simulink model "SimuRISC"  (R2024b)
settings: Solver=FixedStepAuto  StartTime=0.0  StopTime=inf  RelTol=1e-3
values from neighbouring files (symbols this model uses):
  entryPointAddress = hex2dec('80000000')    [initSimuRISC.m]
  modelStopCondition = "tohost"    [initSimuRISC.m]
  tohost_address = hex2dec('1000')    [initSimuRISC.m]
libraries: hdlsllib x18, simulink x2
settings Model: Creator=stefa  LastModifiedBy=stefano
settings OptimizationCC: BlockReduction=off  ConditionallyExecuteInputs=off  DefaultParameterBehavior=Inlined
settings RTWCC: GPUComputeCapability=3.5

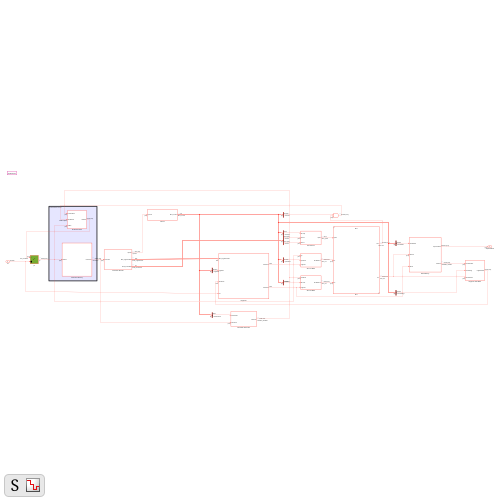
[thumbnail: Simulink's stored preview of the top-level diagram]
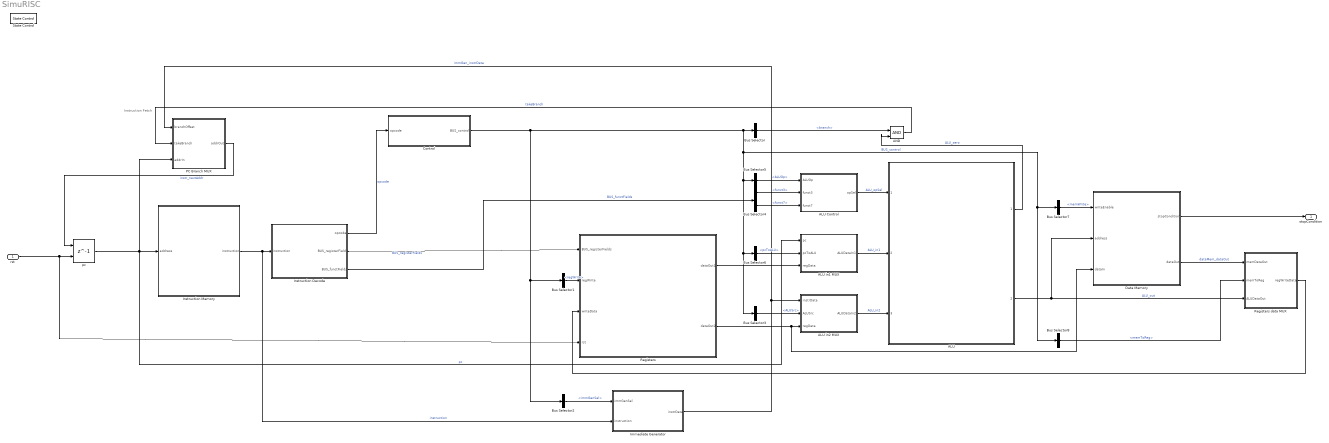
== system SimuRISC ==
  note: Instruction Fetch
  rst : Inport  OutDataTypeStr=boolean
  ALU : Subsystem  ReferencedSubsystem=ALU
  ALU Control : Subsystem
  ALU in1 MUX : Subsystem
  ALU in2 MUX : Subsystem
  AND : Logic  IconShape=distinctive  AllPortsSameDT=off  OutDataTypeStr=boolean
  Bus Selector : BusSelector  OutputSignals=branch
  Bus Selector1 : BusSelector  OutputSignals=regWrite
  Bus Selector2 : BusSelector  OutputSignals=immGenSel
  Bus Selector3 : BusSelector  OutputSignals=ALUSrc
  Bus Selector4 : BusSelector  OutputSignals=funct3,funct7
  Bus Selector5 : BusSelector  OutputSignals=ALUOp
  Bus Selector6 : BusSelector  OutputSignals=pcToALU
  Bus Selector7 : BusSelector  OutputSignals=memWrite
  Bus Selector8 : BusSelector  OutputSignals=memToReg
  Control : Subsystem
  Data Memory : Subsystem
  Immediate Generator : Subsystem
  Instruction Decode : Subsystem
  Instruction Memory : Subsystem
  PC Branch MUX : Subsystem
  Registers : Subsystem
  Registers data MUX : Subsystem
  State Control : StateControl  StateControl=Synchronous
  pc : Delay  DelayLength=1  InitialCondition=entryPointAddress  ExternalReset=Level hold
      settings: InputPortMap=u0,r5
  stopCondition : Outport
  wires:
  pc/1 -> PC Branch MUX/3(addrIn), ALU in1 MUX/1(pc), Instruction Memory/1(address)  "pc"
  PC Branch MUX/1(addrOut) -> pc/1  "instr_nextAddr"
  Immediate Generator/1(instrData) -> ALU in2 MUX/1(instrData), PC Branch MUX/1(branchOffset)  "immGen_instrData"
  AND/1 -> PC Branch MUX/2(takeBranch)  "takeBranch"
  Instruction Memory/1(instruction) -> Immediate Generator/2(instruction), Instruction Decode/1(instruction)  "instruction"
  Instruction Decode/1(opcode) -> Control/1(opcode)  "opcode"
  rst/1 -> Registers/4(rst), pc/2
  Registers/2(dataOut2) -> Data Memory/3(dataIn), ALU in2 MUX/3(regData)
  ALU in2 MUX/1(ALUDataIn2) -> ALU/3  "ALU_in2"
  ALU Control/1(opSel) -> ALU/1  "ALU_opSel"
  ALU/1 -> AND/2  "ALU_zero"
  Control/1(BUS_control) -> Bus Selector1/1, Bus Selector2/1, Bus Selector/1, Bus Selector8/1, Bus Selector7/1, Bus Selector6/1, Bus Selector3/1, Bus Selector5/1  "BUS_control"
  Registers data MUX/1(regWriteData) -> Registers/3(writeData)
  ALU/2 -> Data Memory/2(address), Registers data MUX/3(ALUDataOut)  "ALU_out"
  Data Memory/2(dataOut) -> Registers data MUX/1(memDataOut)  "dataMem_dataOut"
  Bus Selector/1 -> AND/1  "<branch>"
  Instruction Decode/2(BUS_registerFields) -> Registers/1(BUS_registerFields)  "BUS_registerFields"
  Bus Selector1/1 -> Registers/2(regWrite)  "<regWrite>"
  Bus Selector2/1 -> Immediate Generator/1(immGenSel)  "<immGenSel>"
  Bus Selector3/1 -> ALU in2 MUX/2(ALUSrc)  "<ALUSrc>"
  Instruction Decode/3(BUS_functFields) -> Bus Selector4/1  "BUS_functFields"
  Bus Selector4/1 -> ALU Control/2(funct3)  "<funct3>"
  Bus Selector4/2 -> ALU Control/3(funct7)  "<funct7>"
  Bus Selector5/1 -> ALU Control/1(ALUOp)  "<ALUOp>"
  ALU in1 MUX/1(ALUDataIn1) -> ALU/2  "ALU_in1"
  Registers/1(dataOut1) -> ALU in1 MUX/3(regData)
  Bus Selector6/1 -> ALU in1 MUX/2(pcToALU)  "<pcToALU>"
  Bus Selector7/1 -> Data Memory/1(writeEnable)  "<memWrite>"
  Bus Selector8/1 -> Registers data MUX/2(memToReg)  "<memToReg>"
  Data Memory/1(stopCondition) -> stopCondition/1

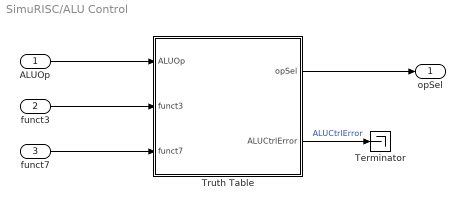
== system SimuRISC/ALU Control ==
  ALUOp : Inport
  funct3 : Inport  Port=2
  funct7 : Inport  Port=3
  Terminator : Terminator
  Truth Table : Truth Table  TreatAsAtomicUnit=on
  opSel : Outport
  wires:
  ALUOp/1 -> Truth Table/1(ALUOp)
  funct3/1 -> Truth Table/2(funct3)
  funct7/1 -> Truth Table/3(funct7)
  Truth Table/1(opSel) -> opSel/1
  Truth Table/2(ALUCtrlError) -> Terminator/1  "ALUCtrlError"

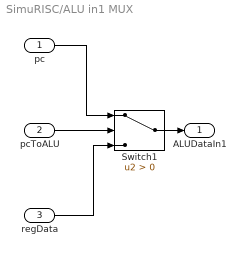
== system SimuRISC/ALU in1 MUX ==
  pc : Inport
  pcToALU : Inport  Port=2
  regData : Inport  Port=3
  Switch1 : Switch  Criteria=u2 > Threshold  SaturateOnIntegerOverflow=off  InputSameDT=off
  ALUDataIn1 : Outport
  wires:
  pc/1 -> Switch1/1
  pcToALU/1 -> Switch1/2
  regData/1 -> Switch1/3
  Switch1/1 -> ALUDataIn1/1

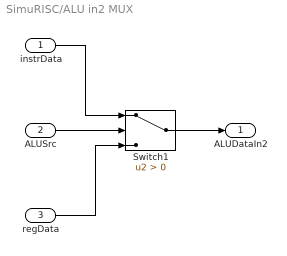
== system SimuRISC/ALU in2 MUX ==
  instrData : Inport
  ALUSrc : Inport  Port=2
  regData : Inport  Port=3
  Switch1 : Switch  Criteria=u2 > Threshold  SaturateOnIntegerOverflow=off  InputSameDT=off
  ALUDataIn2 : Outport
  wires:
  instrData/1 -> Switch1/1
  ALUSrc/1 -> Switch1/2
  regData/1 -> Switch1/3
  Switch1/1 -> ALUDataIn2/1

== system SimuRISC/Control ==
  note: ALUOp : add (00) for loads and stores, subtract and test if zero (01) for beq, or be
      | determined by the operation encoded in the funct7 and funct3 fields
      | (10)
  opcode : Inport
  Bus Creator : BusCreator  Inputs=9
  Opcode Decoder : Truth Table  TreatAsAtomicUnit=on
  BUS_control : Outport
  wires:
  opcode/1 -> Opcode Decoder/1(opcode)
  Opcode Decoder/1(ALUSrc) -> Bus Creator/1
  Opcode Decoder/2(memToReg) -> Bus Creator/2
  Opcode Decoder/3(regWrite) -> Bus Creator/3
  Opcode Decoder/4(memRead) -> Bus Creator/4
  Opcode Decoder/5(memWrite) -> Bus Creator/5
  Opcode Decoder/6(branch) -> Bus Creator/6
  Opcode Decoder/7(ALUOp) -> Bus Creator/7
  Bus Creator/1 -> BUS_control/1
  Opcode Decoder/8(immGenSel) -> Bus Creator/8
  Opcode Decoder/9(pcToALU) -> Bus Creator/9

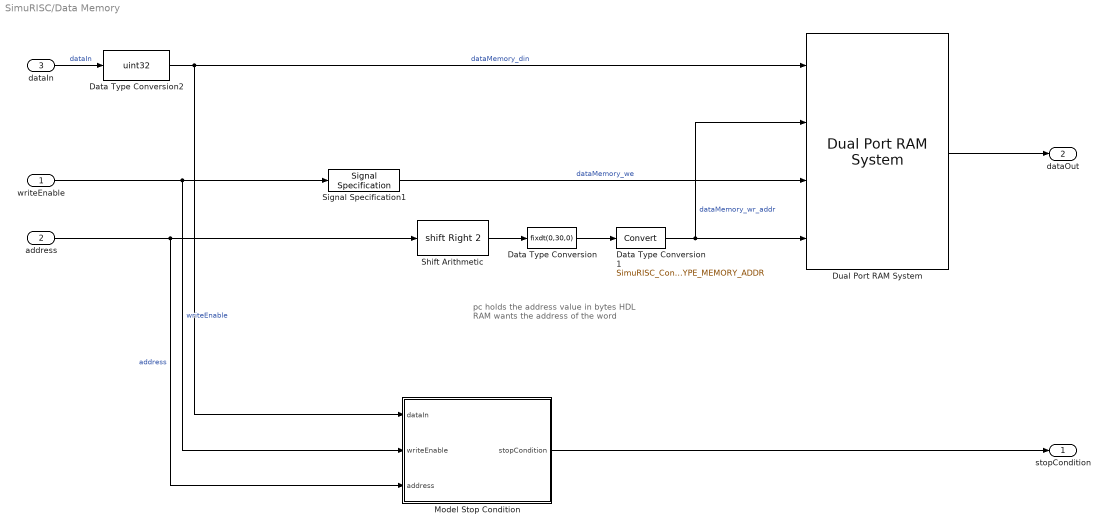
== system SimuRISC/Data Memory ==
  note: pc holds the address value in bytes
      | HDL RAM wants the address of the word
  writeEnable : Inport
  address : Inport  Port=2
  dataIn : Inport  Port=3
  Data Type Conversion : DataTypeConversion  OutDataTypeStr=fixdt(0,30,0)  SaturateOnIntegerOverflow=off  RndMeth=Floor
  Data Type Conversion1 : DataTypeConversion  OutDataTypeStr=SimuRISC_Constants.DATATYPE_MEMORY_ADDR  SaturateOnIntegerOverflow=off  RndMeth=Floor
  Data Type Conversion2 : DataTypeConversion  OutDataTypeStr=uint32  ConvertRealWorld=Stored Integer (SI)  SaturateOnIntegerOverflow=off  RndMeth=Floor
  Dual Port RAM System : hdlsllib/HDL RAMs/Dual Port RAM System  RAMType=Simple dual port  AsyncRead=off  WriteOutputValue=New data  RAMInitialValue=dataMemory  allowBusInputs=off  WritesHaveOutput=on  NumReads=0  NumWrites=1  SimulateUsing=Code generation  ModelRAMDelay=off
  Model Stop Condition : Subsystem  Variant=on  VariantControl=Subsystem  AllowZeroVariantControls=on
  Shift Arithmetic : ArithShift  BitShiftNumber=2  BitShiftDirection=Right
  Signal Specification1 : SignalSpecification  OutDataTypeStr=boolean
  stopCondition : Outport
  dataOut : Outport  Port=2
  wires:
  Data Type Conversion/1 -> Data Type Conversion1/1
  dataIn/1 -> Data Type Conversion2/1  "dataIn"
  Dual Port RAM System/1 -> dataOut/1
  Data Type Conversion1/1 -> Dual Port RAM System/2, Dual Port RAM System/4  "dataMemory_wr_addr"
  writeEnable/1 -> Signal Specification1/1, Model Stop Condition/2(writeEnable)  "writeEnable"
  Shift Arithmetic/1 -> Data Type Conversion/1
  address/1 -> Shift Arithmetic/1, Model Stop Condition/3(address)  "address"
  Signal Specification1/1 -> Dual Port RAM System/3  "dataMemory_we"
  Data Type Conversion2/1 -> Dual Port RAM System/1, Model Stop Condition/1(dataIn)  "dataMemory_din"
  Model Stop Condition/1(stopCondition) -> stopCondition/1

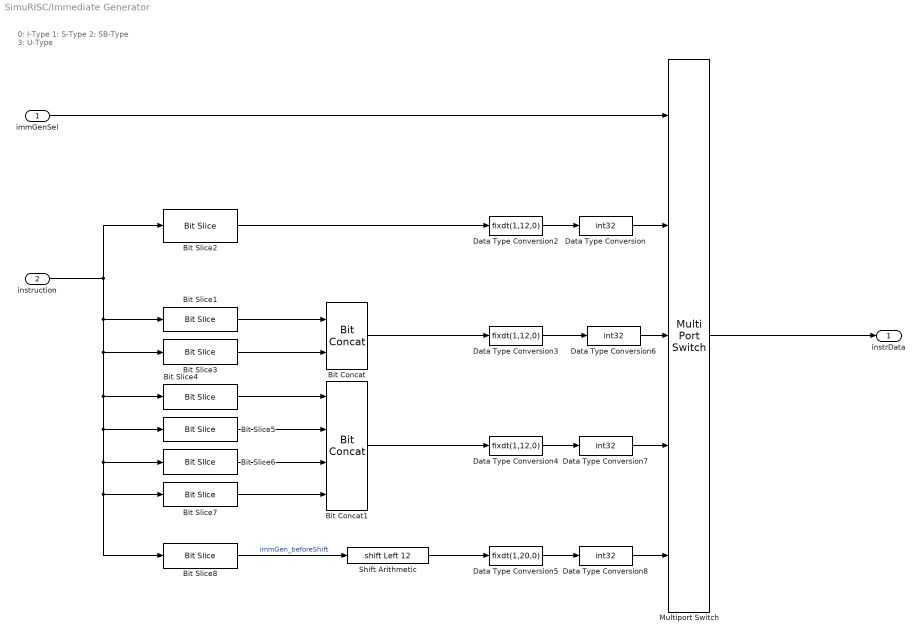
== system SimuRISC/Immediate Generator ==
  note: 0: I-Type
      | 1: S-Type
      | 2: SB-Type
      | 3: U-Type
  immGenSel : Inport
  instruction : Inport  Port=2
  Bit Concat : hdlsllib/Logic and Bit Operations/Bit Concat  numInputs=2
  Bit Concat1 : hdlsllib/Logic and Bit Operations/Bit Concat  numInputs=4
  Bit Slice1 : hdlsllib/Logic and Bit Operations/Bit Slice  lidx=31  ridx=25
  Bit Slice2 : hdlsllib/Logic and Bit Operations/Bit Slice  lidx=31  ridx=20
  Bit Slice3 : hdlsllib/Logic and Bit Operations/Bit Slice  lidx=11  ridx=7
  Bit Slice4 : hdlsllib/Logic and Bit Operations/Bit Slice  lidx=31  ridx=31
  Bit Slice5 : hdlsllib/Logic and Bit Operations/Bit Slice  lidx=7  ridx=7
  Bit Slice6 : hdlsllib/Logic and Bit Operations/Bit Slice  lidx=30  ridx=25
  Bit Slice7 : hdlsllib/Logic and Bit Operations/Bit Slice  lidx=11  ridx=8
  Bit Slice8 : hdlsllib/Logic and Bit Operations/Bit Slice  lidx=31  ridx=12
  Data Type Conversion{,6..8} (4 alike) : DataTypeConversion  OutDataTypeStr=int32  SaturateOnIntegerOverflow=off  RndMeth=Floor
  Data Type Conversion2 : DataTypeConversion  OutDataTypeStr=fixdt(1,12,0)  ConvertRealWorld=Stored Integer (SI)  SaturateOnIntegerOverflow=off  RndMeth=Floor
  Data Type Conversion3 : DataTypeConversion  OutDataTypeStr=fixdt(1,12,0)  ConvertRealWorld=Stored Integer (SI)  SaturateOnIntegerOverflow=off  RndMeth=Floor
  Data Type Conversion4 : DataTypeConversion  OutDataTypeStr=fixdt(1,12,0)  ConvertRealWorld=Stored Integer (SI)  SaturateOnIntegerOverflow=off  RndMeth=Floor
  Data Type Conversion5 : DataTypeConversion  OutDataTypeStr=fixdt(1,20,0)  ConvertRealWorld=Stored Integer (SI)  SaturateOnIntegerOverflow=off  RndMeth=Floor
  Multiport Switch : MultiPortSwitch  DataPortOrder=Zero-based contiguous  Inputs=4  DiagnosticForDefault=Warning  zeroidx=on  SaturateOnIntegerOverflow=off  InputSameDT=off
  Shift Arithmetic : ArithShift  BitShiftNumber=12  BitShiftDirection=Left
  instrData : Outport
  wires:
  Bit Slice2/1 -> Data Type Conversion2/1
  Bit Slice1/1 -> Bit Concat/1
  Bit Slice3/1 -> Bit Concat/2
  instruction/1 -> Bit Slice4/1, Bit Slice5/1, Bit Slice8/1, Bit Slice7/1, Bit Slice6/1, Bit Slice3/1, Bit Slice1/1, Bit Slice2/1
  Bit Concat/1 -> Data Type Conversion3/1
  Bit Concat1/1 -> Data Type Conversion4/1
  Multiport Switch/1 -> instrData/1
  Bit Slice4/1 -> Bit Concat1/1
  Bit Slice5/1 -> Bit Concat1/2
  Bit Slice6/1 -> Bit Concat1/3
  Bit Slice7/1 -> Bit Concat1/4
  Bit Slice8/1 -> Shift Arithmetic/1  "immGen_beforeShift"
  Shift Arithmetic/1 -> Data Type Conversion5/1
  immGenSel/1 -> Multiport Switch/1
  Data Type Conversion/1 -> Multiport Switch/2
  Data Type Conversion2/1 -> Data Type Conversion/1
  Data Type Conversion3/1 -> Data Type Conversion6/1
  Data Type Conversion4/1 -> Data Type Conversion7/1
  Data Type Conversion5/1 -> Data Type Conversion8/1
  Data Type Conversion6/1 -> Multiport Switch/3
  Data Type Conversion7/1 -> Multiport Switch/4
  Data Type Conversion8/1 -> Multiport Switch/5

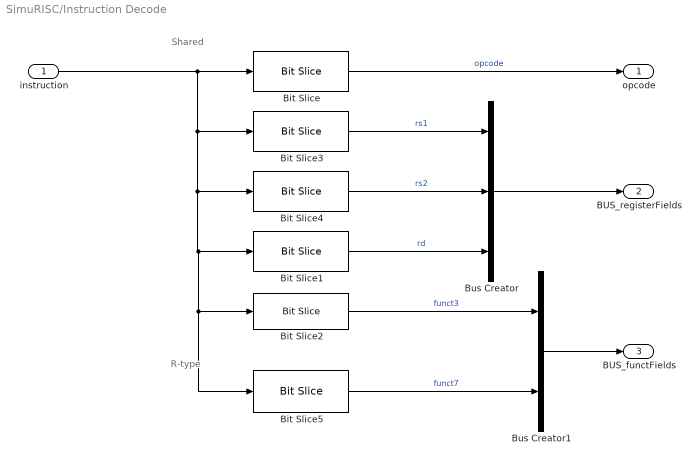
== system SimuRISC/Instruction Decode ==
  note: Shared
  note: R-type
  instruction : Inport
  Bit Slice : hdlsllib/Logic and Bit Operations/Bit Slice  lidx=6  ridx=0
  Bit Slice1 : hdlsllib/Logic and Bit Operations/Bit Slice  lidx=11  ridx=7
  Bit Slice2 : hdlsllib/Logic and Bit Operations/Bit Slice  lidx=14  ridx=12
  Bit Slice3 : hdlsllib/Logic and Bit Operations/Bit Slice  lidx=19  ridx=15
  Bit Slice4 : hdlsllib/Logic and Bit Operations/Bit Slice  lidx=24  ridx=20
  Bit Slice5 : hdlsllib/Logic and Bit Operations/Bit Slice  lidx=31  ridx=25
  Bus Creator : BusCreator  Inputs=3
  Bus Creator1 : BusCreator  Inputs=2
  opcode : Outport
  BUS_registerFields : Outport  Port=2
  BUS_functFields : Outport  Port=3
  wires:
  Bit Slice/1 -> opcode/1  "opcode"
  Bit Slice1/1 -> Bus Creator/3  "rd"
  Bit Slice2/1 -> Bus Creator1/1  "funct3"
  Bit Slice3/1 -> Bus Creator/1  "rs1"
  Bit Slice4/1 -> Bus Creator/2  "rs2"
  Bit Slice5/1 -> Bus Creator1/2  "funct7"
  instruction/1 -> Bit Slice2/1, Bit Slice5/1, Bit Slice1/1, Bit Slice4/1, Bit Slice3/1, Bit Slice/1
  Bus Creator/1 -> BUS_registerFields/1
  Bus Creator1/1 -> BUS_functFields/1

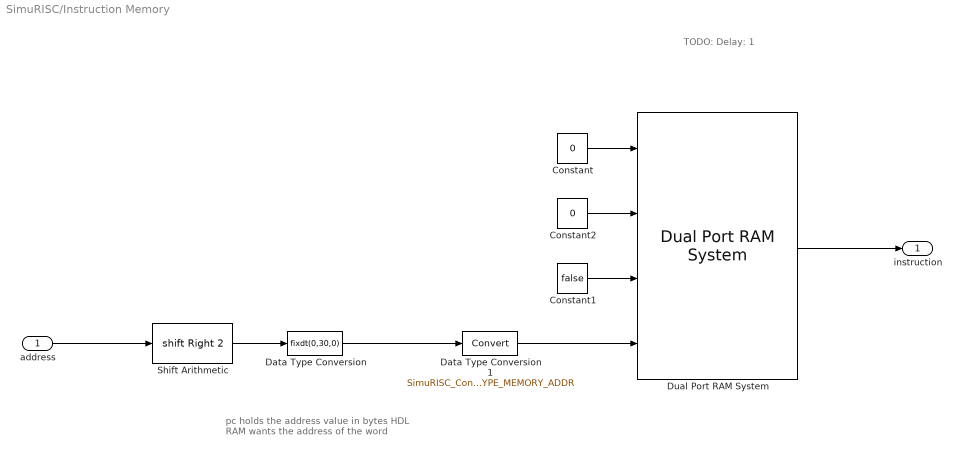
== system SimuRISC/Instruction Memory ==
  note: TODO: Delay: 1
  note: pc holds the address value in bytes
      | HDL RAM wants the address of the word
  address : Inport
  Constant : Constant  Value=0  OutDataTypeStr=uint32  SampleTime=-1
  Constant1 : Constant  Value=false  SampleTime=-1
  Constant2 : Constant  Value=0  OutDataTypeStr=SimuRISC_Constants.DATATYPE_MEMORY_ADDR  SampleTime=-1  LockScale=on
  Data Type Conversion : DataTypeConversion  OutDataTypeStr=fixdt(0,30,0)  SaturateOnIntegerOverflow=off  RndMeth=Floor
  Data Type Conversion1 : DataTypeConversion  OutDataTypeStr=SimuRISC_Constants.DATATYPE_MEMORY_ADDR  SaturateOnIntegerOverflow=off  RndMeth=Floor
  Dual Port RAM System : hdlsllib/HDL RAMs/Dual Port RAM System  RAMType=Simple dual port  AsyncRead=off  WriteOutputValue=New data  RAMInitialValue=instructionMemory  allowBusInputs=off  WritesHaveOutput=on  NumReads=0  NumWrites=1  SimulateUsing=Code generation  ModelRAMDelay=off
  Shift Arithmetic : ArithShift  BitShiftNumber=2  BitShiftDirection=Right
  instruction : Outport
  wires:
  Constant/1 -> Dual Port RAM System/1
  Constant1/1 -> Dual Port RAM System/3
  address/1 -> Shift Arithmetic/1
  Constant2/1 -> Dual Port RAM System/2
  Dual Port RAM System/1 -> instruction/1
  Shift Arithmetic/1 -> Data Type Conversion/1
  Data Type Conversion/1 -> Data Type Conversion1/1
  Data Type Conversion1/1 -> Dual Port RAM System/4

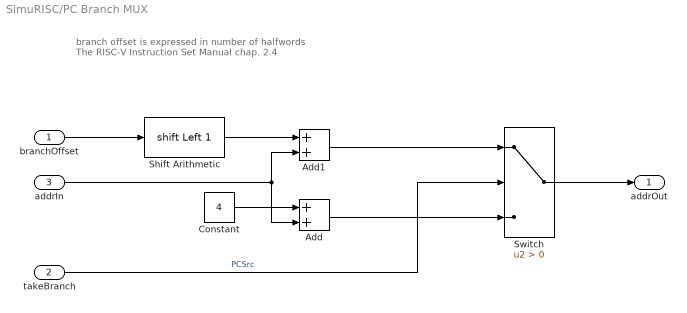
== system SimuRISC/PC Branch MUX ==
  note: branch offset is expressed in number of halfwords
      | The RISC-V Instruction Set Manual chap. 2.4
  branchOffset : Inport
  takeBranch : Inport  Port=2
  addrIn : Inport  Port=3
  Add : Sum  OutDataTypeStr=Inherit: Same as first input
  Add1 : Sum  OutDataTypeStr=Inherit: Same as first input
  Constant : Constant  Value=4  OutDataTypeStr=registerSize  SampleTime=-1
  Shift Arithmetic : ArithShift  BitShiftNumber=1  BitShiftDirection=Left
  Switch : Switch  Criteria=u2 > Threshold  SaturateOnIntegerOverflow=off  InputSameDT=off
  addrOut : Outport
  wires:
  Add/1 -> Switch/3
  addrIn/1 -> Add1/2, Add/2
  Switch/1 -> addrOut/1
  Add1/1 -> Switch/1
  takeBranch/1 -> Switch/2  "PCSrc"
  Constant/1 -> Add/1
  branchOffset/1 -> Shift Arithmetic/1
  Shift Arithmetic/1 -> Add1/1

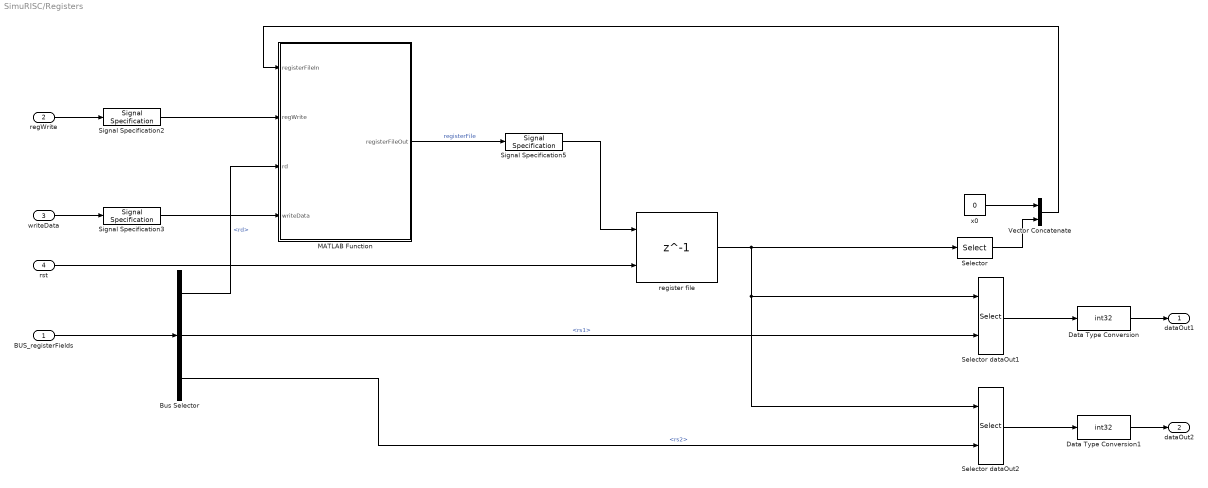
== system SimuRISC/Registers ==
  BUS_registerFields : Inport
  regWrite : Inport  Port=2
  writeData : Inport  Port=3
  rst : Inport  Port=4
  Bus Selector : BusSelector  OutputSignals=rd,rs1,rs2
  Data Type Conversion : DataTypeConversion  OutDataTypeStr=int32  ConvertRealWorld=Stored Integer (SI)  SaturateOnIntegerOverflow=off  RndMeth=Floor
  Data Type Conversion1 : DataTypeConversion  OutDataTypeStr=int32  ConvertRealWorld=Stored Integer (SI)  SaturateOnIntegerOverflow=off  RndMeth=Floor
  MATLAB Function : MATLAB Function  TreatAsAtomicUnit=on
  Selector : Selector  InputPortWidth=32  IndexOptions=Index vector (dialog)  Indices=2:32  OutputSizes=1
  Selector dataOut1 : Selector  IndexMode=Zero-based  InputPortWidth=32  IndexOptions=Index vector (port)  Indices=[1 3]  OutputSizes=1
  Selector dataOut2 : Selector  IndexMode=Zero-based  InputPortWidth=32  IndexOptions=Index vector (port)  Indices=[1 3]  OutputSizes=1
  Signal Specification2 : SignalSpecification  OutDataTypeStr=boolean
  Signal Specification3 : SignalSpecification  OutDataTypeStr=uint32
  Signal Specification5 : SignalSpecification  OutDataTypeStr=uint32  Dimensions=32
  Vector Concatenate : Concatenate
  register file : Delay  DelayLength=1  InitialCondition=uint32(zeros(32,1))  ExternalReset=Level hold
      settings: InputPortMap=u0,r5
  x0 : Constant  Value=0  OutDataTypeStr=registerSize  SampleTime=-1
  dataOut1 : Outport
  dataOut2 : Outport  Port=2
  wires:
  register file/1 -> Selector dataOut1/1, Selector dataOut2/1, Selector/1
  Selector dataOut1/1 -> Data Type Conversion/1
  Selector dataOut2/1 -> Data Type Conversion1/1
  BUS_registerFields/1 -> Bus Selector/1
  rst/1 -> register file/2
  Selector/1 -> Vector Concatenate/2
  x0/1 -> Vector Concatenate/1
  Bus Selector/3 -> Selector dataOut2/2  "<rs2>"
  regWrite/1 -> Signal Specification2/1
  writeData/1 -> Signal Specification3/1
  Signal Specification3/1 -> MATLAB Function/4(writeData)
  MATLAB Function/1(registerFileOut) -> Signal Specification5/1  "registerFile"
  Vector Concatenate/1 -> MATLAB Function/1(registerFileIn)
  Bus Selector/1 -> MATLAB Function/3(rd)  "<rd>"
  Signal Specification2/1 -> MATLAB Function/2(regWrite)
  Signal Specification5/1 -> register file/1
  Bus Selector/2 -> Selector dataOut1/2  "<rs1>"
  Data Type Conversion/1 -> dataOut1/1
  Data Type Conversion1/1 -> dataOut2/1

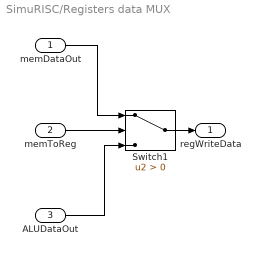
== system SimuRISC/Registers data MUX ==
  memDataOut : Inport
  memToReg : Inport  Port=2
  ALUDataOut : Inport  Port=3
  Switch1 : Switch  Criteria=u2 > Threshold  SaturateOnIntegerOverflow=off  InputSameDT=off
  regWriteData : Outport
  wires:
  memDataOut/1 -> Switch1/1
  memToReg/1 -> Switch1/2
  ALUDataOut/1 -> Switch1/3
  Switch1/1 -> regWriteData/1

== system SimuRISC/Data Memory/Model Stop Condition ==
  dataIn : Inport
  writeEnable : Inport  Port=2
  address : Inport  Port=3
  tohost : Subsystem  VariantControl="strcmp(modelStopCondition, \"tohost\")"
  stopCondition : Outport

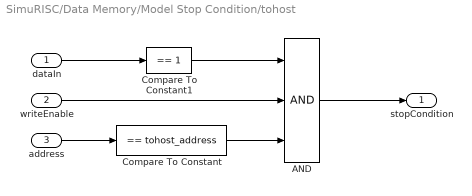
== system SimuRISC/Data Memory/Model Stop Condition/tohost ==
  dataIn : Inport
  writeEnable : Inport  Port=2
  address : Inport  Port=3
  AND : Logic  Inputs=3  IconShape=distinctive  AllPortsSameDT=off  OutDataTypeStr=boolean
  Compare To Constant : simulink/Logic and Bit Operations/Compare To Constant  relop===  const=tohost_address  OutDataTypeStr=boolean
  Compare To Constant1 : simulink/Logic and Bit Operations/Compare To Constant  relop===  const=1  OutDataTypeStr=boolean
  stopCondition : Outport
  wires:
  Compare To Constant/1 -> AND/3
  Compare To Constant1/1 -> AND/1
  address/1 -> Compare To Constant/1
  AND/1 -> stopCondition/1
  dataIn/1 -> Compare To Constant1/1
  writeEnable/1 -> AND/2

== matlab function SimuRISC/Registers/MATLAB Function ==
  data: registerFileIn input; regWrite input; rd input; registerFileOut output; writeData input
 function registerFileOut = registerWrite(registerFileIn, regWrite, rd, writeData)
    registerFileInt = registerFileIn;
    if regWrite
        registerFileInt(rd+1) = writeData;
    end
    registerFileOut = registerFileInt;

== matlab function SimuRISC/ALU Control/Truth Table ==
  data: ALUOp input; opSel output; funct3 input; funct7 input; ALUCtrlError output boolean
function [opSel, ALUCtrlError] = fcn(ALUOp, funct3, funct7)

aVarTruthTableCondition_1 = false;
aVarTruthTableCondition_2 = false;
aVarTruthTableCondition_3 = false;
aVarTruthTableCondition_4 = false;
aVarTruthTableCondition_5 = false;
aVarTruthTableCondition_6 = false;
aVarTruthTableCondition_7 = false;


% lw;sw;lui

aVarTruthTableCondition_1 = logical(ALUOp == 0);

% beq

aVarTruthTableCondition_2 = logical(ALUOp == 1);

% R-Type

aVarTruthTableCondition_3 = logical(ALUOp == 2);

% R-Type: add

aVarTruthTableCondition_4 = logical(funct7 == 0 && funct3 == 0);

% R-Type: sub

aVarTruthTableCondition_5 = logical(funct7 == 32 && funct3 == 0);

% R-Type: AND

aVarTruthTableCondition_6 = logical(funct7 == 0 && funct3 == 7);

% R-Type: OR

aVarTruthTableCondition_7 = logical(funct7 == 0 && funct3 == 6);

if (aVarTruthTableCondition_1 && ~aVarTruthTableCondition_2 && ~aVarTruthTableCondition_3)
    add();
elseif (~aVarTruthTableCondition_1 && aVarTruthTableCondition_2 && ~aVarTruthTableCondition_3)
    sub();
elseif (~aVarTruthTableCondition_1 && ~aVarTruthTableCondition_2 && aVarTruthTableCondition_3 && aVarTruthTableCondition_4)
    add();
elseif (~aVarTruthTableCondition_1 && ~aVarTruthTableCondition_2 && aVarTruthTableCondition_3 && aVarTruthTableCondition_5)
    sub();
elseif (~aVarTruthTableCondition_1 && ~aVarTruthTableCondition_2 && aVarTruthTableCondition_3 && aVarTruthTableCondition_6)
    and();
elseif (~aVarTruthTableCondition_1 && ~aVarTruthTableCondition_2 && aVarTruthTableCondition_3 && aVarTruthTableCondition_7)
    or();
else % Default
    DA();
end

function DA()

% default action (should never reach)

ALUCtrlError = true;
opSel = 15;

function and()

% and

opSel = 0;
ALUCtrlError = false;

function or()

% or

opSel = 1;
ALUCtrlError = false;

function add()

% add

opSel = 2;
ALUCtrlError = false;

function sub()

% sub

opSel = 3;
ALUCtrlError = false;

== matlab function SimuRISC/Control/Opcode Decoder ==
  data: opcode input; ALUSrc output boolean; memToReg output boolean; regWrite output boolean; memRead output boolean; memWrite output boolean; branch output boolean; ALUOp output fixdt(0,2,0); immGenSel output uint8; pcToALU output boolean
function [ALUSrc, memToReg, regWrite, memRead, memWrite, branch, ALUOp, immGenSel, pcToALU] = fcn(opcode)

aVarTruthTableCondition_1 = false;
aVarTruthTableCondition_2 = false;
aVarTruthTableCondition_3 = false;
aVarTruthTableCondition_4 = false;
aVarTruthTableCondition_5 = false;
aVarTruthTableCondition_6 = false;
aVarTruthTableCondition_7 = false;


% R-Type

aVarTruthTableCondition_1 = logical(opcode == 51);

% I-Type - Memory Load

aVarTruthTableCondition_2 = logical(opcode == 3);

% I-Type - Arithmetical

aVarTruthTableCondition_3 = logical(opcode == 19);

% S-Type

aVarTruthTableCondition_4 = logical(opcode == 35);

% SB-Type

aVarTruthTableCondition_5 = logical(opcode == 99);

% U-Type - LUI

aVarTruthTableCondition_6 = logical(opcode == 55);

% U-Type - AUIPC

aVarTruthTableCondition_7 = logical(opcode == 23);

if (aVarTruthTableCondition_1)
    R();
elseif (aVarTruthTableCondition_2)
    I_load();
elseif (aVarTruthTableCondition_3)
    I_arithm();
elseif (aVarTruthTableCondition_4)
    S();
elseif (aVarTruthTableCondition_5)
    SB();
elseif (aVarTruthTableCondition_6)
    U_LUI();
elseif (aVarTruthTableCondition_7)
    U_AUIPC();
else % Default
    DA();
end

function DA()

% default action (should never reach)

ALUSrc = false;
memToReg = false;
regWrite = false;
memRead = false;
memWrite = false;
branch = false;
ALUOp = 3;
immGenSel = 0;
pcToALU = false;

function R()

% R-Type

ALUSrc = false;
memToReg = false;
regWrite = true;
memRead = false;
memWrite = false;
branch = false;
ALUOp = 2;
immGenSel = 0;
pcToALU = false;

function I_load()

% I-Type - Memory Load

ALUSrc = true;
memToReg = true;
regWrite = true;
memRead = true;
memWrite = false;
branch = false;
ALUOp = 0;
immGenSel = 0;
pcToALU = false;

function I_arithm()

% I-Type - Arithmetical

ALUSrc = true;
memToReg = false;
regWrite = true;
memRead = false;
memWrite = false;
branch = false;
ALUOp = 0;
immGenSel = 0;
pcToALU = false;

function S()

% S -Type

ALUSrc = true;
memToReg = false;
regWrite = false;
memRead = false;
memWrite = true;
branch = false;
ALUOp = 0;
immGenSel = 1;
pcToALU = false;

function SB()

% SB-Type

ALUSrc = false;
memToReg = false;
regWrite = false;
memRead = false;
memWrite = false;
branch = true;
ALUOp = 1;
immGenSel = 2;
pcToALU = false;

function U_LUI()

% U-Type - LUI

ALUSrc = true;
memToReg = false;
regWrite = true;
memRead = false;
memWrite = false;
branch = false;
ALUOp = 0;
immGenSel = 3;
pcToALU = false;

function U_AUIPC()

% U-Type - AUIPC

ALUSrc = true;
memToReg = false;
regWrite = true;
memRead = false;
memWrite = false;
branch = false;
ALUOp = 0;
immGenSel = 3;
pcToALU = true;
